simulink model "sample1_controler"  (R2021a)
settings: Solver=FixedStepAuto  StartTime=0.0  StopTime=20  FixedStep=0.01  RelTol=1e-3
settings Model: Creator=Davie  LastModifiedBy=Davie

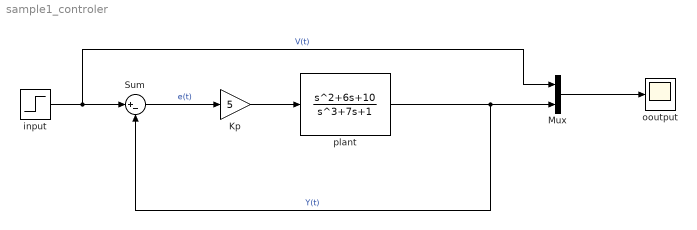
== system sample1_controler ==
  Kp : Gain  Gain=5
  Mux : Mux  Inputs=2
  Sum : Sum  Inputs=|+-
  input : Step  SampleTime=0
  ooutput : Scope
  plant : TransferFcn  Numerator=[1 6 10]  Denominator=[1 0 7 1]
  wires:
  plant/1 -> Mux/2, Sum/2  "Y(t)"
  Sum/1 -> Kp/1  "e(t)"
  input/1 -> Mux/1, Sum/1  "V(t)"
  Kp/1 -> plant/1
  Mux/1 -> ooutput/1
